simulink model "fig_5_2_12"  (R2014b)
settings: Solver=ode23tb  StartTime=0.0  StopTime=0.005  FixedStep=1e-5  RelTol=1e-4
undefined symbols (not defined in the file): Ts
libraries: powerlib x9
settings Model: Creator=umi  LastModifiedBy=umi
settings DebuggingCC: UnconnectedInputMsg=none  UnconnectedOutputMsg=none  UnconnectedLineMsg=none

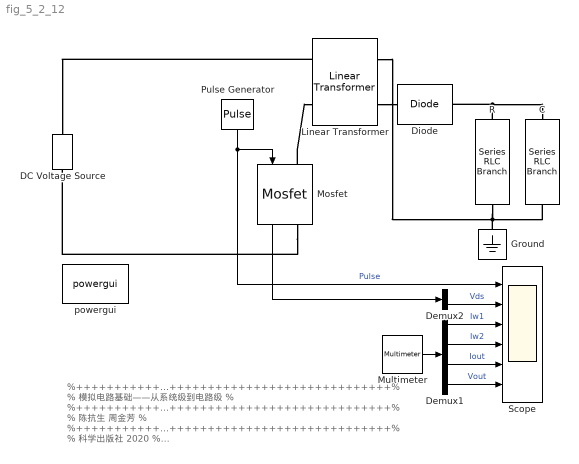
== system fig_5_2_12 ==
  note: %++++++++++++++++++++++++++++++++++++++++%
      | % 模拟电路基础——从系统级到电路级 %
      | %++++++++++++++++++++++++++++++++++++++++%
      | % 陈抗生 周金芳 %
      | %++++++++++++++++++++++++++++++++++++++++%
      | % 科学出版社 2020 %
      | %++++++++++++++++++++++++++++++++++++++++%
  "C " : powerlib/Elements/Series RLC Branch  LConnTagsString=__new0  RConnTagsString=__new0  BranchType=C  Resistance=1  Inductance=1e-3  SetiL0=off  InitialCurrent=0  Capacitance=1000e-6  Setx0=off  InitialVoltage=0  Measurements=Branch voltage
  DC Voltage Source : powerlib/Electrical Sources/DC Voltage Source  Amplitude=100  Measurements=None
  Demux1 : Demux
  Demux2 : Demux  Outputs=2
  Diode : powerlib/Power Electronics/Diode  Ron=0.05  Lon=1e-8  Vf=0.7  IC=0  UseSnubber=off  Rs=1e5  Cs=Inf  Measurements=off
  Ground : powerlib/Elements/Ground  LConnTagsString=a
  Linear Transformer : powerlib/Elements/Linear Transformer  UNITS=SI  NominalPower=[250e6 60]  winding1=[100 0 0]  winding2=[20 0 0]  ThreeWindings=off  winding3=[3.15e+05 0.7938 0.084223]  RmLm=[Inf 500e-6]  Measurements=Winding currents  DataType=on
  Mosfet : powerlib/Power Electronics/Mosfet  Ron=0.1  Lon=0  Rd=0.01  Vfd=0  IC=0  Rs=1e5  Cs=inf  Measurements=on
  Multimeter : powerlib/Measurements/Multimeter  PhasorSimulation=off  OutputType=Complex  sel=[3 4 2 1]  L=4  Gain=[1 1 1 1]  yselected={'Iw1: Linear Transformer','Iw2: Linear Transformer','Ib: R ','Ub: C '};  PSBOutputType=1  PSBequivalent=0  AxesSetting=[0,0.1,-100,100]  Display=0  SavedBlockNames=-11
  Pulse Generator : DiscretePulseGenerator  PulseType=Time based  Period=1e-4  PulseWidth=50
  "R " : powerlib/Elements/Series RLC Branch  LConnTagsString=__new0  RConnTagsString=__new0  BranchType=R  Resistance=1  Inductance=1e-3  SetiL0=off  InitialCurrent=0  Capacitance=1e-6  Setx0=off  InitialVoltage=0  Measurements=Branch current
  Scope : Scope  NumInputPorts=6
      settings: TimeRange=0.005  YMin=-1~-50~-5~-50~-5~-5  YMax=2~250~15~100~5~5  MaxDataPoints=7000
  powergui : powerlib/powergui  Priority=1  SimulationMode=Continuous  SolverType=Tustin/Backward Euler (TBE)  SampleTime=Ts  frequency=60  SPID=on  DisableSnubberDevices=on  DisableRonSwitches=off  DisableVfSwitches=off  SwTol=0  DisplayEquations=off  Interpol=off  methode=off  Ts=100  frequencyindice=0  Pbase=100e6  ErrMax=1e-4  Iterations=50  UnitsV=kV  UnitsW=MW  FunctionMessages=off  echomessages=off  HookPort=off  EnableUseOfTLC=off  x0status=blocks  RestoreLinks=warning  ResistiveCurrentMeasurement=off  Frange=[0:2:500]  Ylog=off  Xlog=on  ShowGrid=off  save=off  variable=ZData  structure=0  ZoomFFT=off  StartTime=0.0  cycles=1  DisplayStyle=1  fundamental=60  FreqAxis=off  MaxFrequency=1000  frequencyindicesteady=1  RmsSteady=1  display=off
  wires:
  Pulse Generator/1 -> Mosfet/1, Scope/1  "Pulse"
  Mosfet/1 -> Demux2/1
  Multimeter/1 -> Demux1/1
  Demux2/2 -> Scope/2  "Vds"
  Demux1/1 -> Scope/3  "Iw1"
  Demux1/2 -> Scope/4  "Iw2"
  Demux1/3 -> Scope/5  "Iout"
  Demux1/4 -> Scope/6  "Vout"
  connections:
  Mosfet/RConn1 -- DC Voltage Source/LConn1
  Mosfet/LConn1 -- Linear Transformer/LConn2
  Linear Transformer/LConn1 -- DC Voltage Source/RConn1
  Linear Transformer/RConn2 -- Diode/LConn1
  "R "/RConn1 -- Linear Transformer/RConn1 -- "C "/RConn1 -- Ground/LConn1
  "R "/LConn1 -- Diode/RConn1 -- "C "/LConn1
